simulink model "Solar_pressure_on_10_faces"  (R2023b)
settings: Solver=VariableStepAuto  StartTime=0.0  StopTime=10.0  RelTol=1e-3
undefined symbols (not defined in the file or in its folder): A_1, A_10, A_2, A_3, A_4, A_5, A_6, A_7, A_8, A_9, N_1, N_10, N_2, N_3, N_4, N_5, N_6, N_7, N_8, N_9, r_1, r_10, r_2, r_3, r_4, r_5, r_6, r_7, r_8, r_9, rho_d1, rho_d10, rho_d2, rho_d3, rho_d4, rho_d5, rho_d6, rho_d7, rho_d8, rho_d9, rho_s1, rho_s10, rho_s2, rho_s3, rho_s4, rho_s5, rho_s6, rho_s7, rho_s8, rho_s9
libraries: matrix_library x10
settings Model: Creator=rkomiii_masca  LastModifiedBy=rkomiii_masca

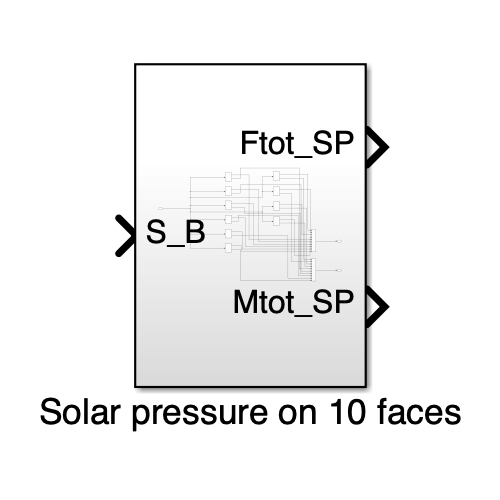
[thumbnail: Simulink's stored preview of the top-level diagram]
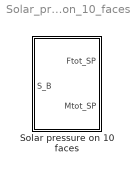
== system Solar_pressure_on_10_faces ==
  Solar pressure on 10 faces : Subsystem

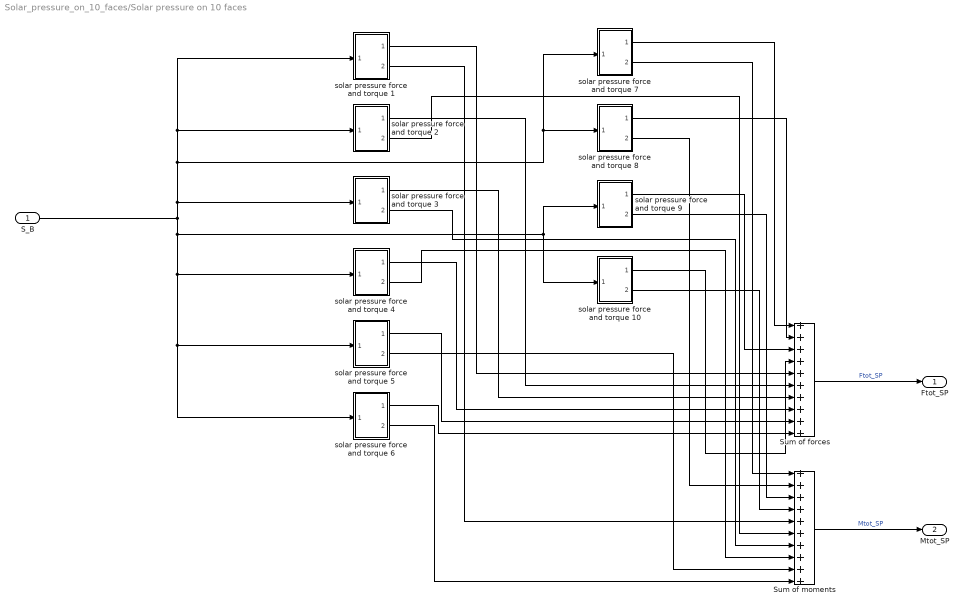
== system Solar_pressure_on_10_faces/Solar pressure on 10 faces ==
  S_B : Inport
  Sum of forces : Sum  Inputs=++++++++++
  Sum of moments : Sum  Inputs=++++++++++
  solar pressure force and torque 1 : Subsystem
  solar pressure force and torque 10 : Subsystem
  solar pressure force and torque 2 : Subsystem
  solar pressure force and torque 3 : Subsystem
  solar pressure force and torque 4 : Subsystem
  solar pressure force and torque 5 : Subsystem
  solar pressure force and torque 6 : Subsystem
  solar pressure force and torque 7 : Subsystem
  solar pressure force and torque 8 : Subsystem
  solar pressure force and torque 9 : Subsystem
  Ftot_SP : Outport
  Mtot_SP : Outport  Port=2
  wires:
  solar pressure force and torque 1/1(F_1) -> Sum of forces/5
  solar pressure force and torque 2/1(F_2) -> Sum of forces/6
  solar pressure force and torque 3/1(F_3) -> Sum of forces/7
  solar pressure force and torque 4/1(F_4) -> Sum of forces/8
  solar pressure force and torque 5/1(F_5) -> Sum of forces/9
  solar pressure force and torque 6/1(F_6) -> Sum of forces/10
  solar pressure force and torque 7/1(F_7) -> Sum of forces/1
  solar pressure force and torque 8/1(F_8) -> Sum of forces/2
  solar pressure force and torque 9/1(F_9) -> Sum of forces/3
  solar pressure force and torque 10/1(F_10) -> Sum of forces/4
  solar pressure force and torque 1/2(M_1) -> Sum of moments/5
  solar pressure force and torque 2/2(M_2) -> Sum of moments/6
  solar pressure force and torque 3/2(M_3) -> Sum of moments/7
  solar pressure force and torque 4/2(M_4) -> Sum of moments/8
  solar pressure force and torque 5/2(M_5) -> Sum of moments/9
  solar pressure force and torque 6/2(M_6) -> Sum of moments/10
  solar pressure force and torque 7/2(M_7) -> Sum of moments/1
  solar pressure force and torque 8/2(M_8) -> Sum of moments/2
  solar pressure force and torque 9/2(M_9) -> Sum of moments/3
  solar pressure force and torque 10/2(M_10) -> Sum of moments/4
  Sum of forces/1 -> Ftot_SP/1  "Ftot_SP"
  Sum of moments/1 -> Mtot_SP/1  "Mtot_SP"
  S_B/1 -> solar pressure force and torque 10/1(s_B), solar pressure force and torque 9/1(s_B), solar pressure force and torque 6/1(s_B), solar pressure force and torque 5/1(s_B), solar pressure force and torque 4/1(s_B), solar pressure force and torque 7/1(s_B), solar pressure force and torque 8/1(s_B), solar pressure force and torque 1/1(s_B), solar pressure force and torque 2/1(s_B), solar pressure force and torque 3/1(s_B)

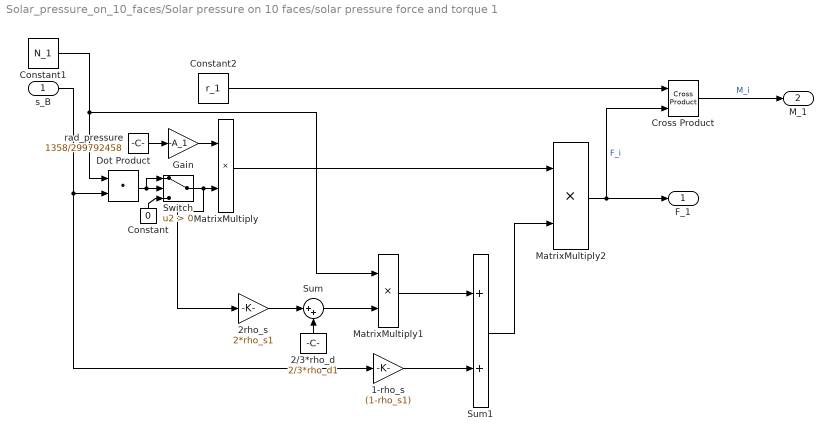
== system Solar_pressure_on_10_faces/Solar pressure on 10 faces/solar pressure force and torque 1 ==
  s_B : Inport
  1-rho_s : Gain  Gain=(1-rho_s1)
  2/3*rho_d : Constant  Value=2/3*rho_d1
  2rho_s : Gain  Gain=2*rho_s1
  Constant : Constant  Value=0
  Constant1 : Constant  Value=N_1
  Constant2 : Constant  Value=r_1
  Cross Product : matrix_library/Cross Product
  Dot Product : DotProduct  OutDataTypeStr=Inherit: Inherit via internal rule
  Gain : Gain  Gain=-A_1
  MatrixMultiply : Product
  MatrixMultiply1 : Product
  MatrixMultiply2 : Product
  Sum : Sum  Inputs=|++
  Sum1 : Sum
  Switch : Switch  Criteria=u2 > Threshold  SaturateOnIntegerOverflow=off  InputSameDT=off
  rad_pressure : Constant  Value=1358/299792458
  F_1 : Outport
  M_1 : Outport  Port=2
  wires:
  MatrixMultiply2/1 -> Cross Product/2, F_1/1  "F_i"
  MatrixMultiply/1 -> MatrixMultiply2/1
  Sum1/1 -> MatrixMultiply2/2
  s_B/1 -> 1-rho_s/1, Dot Product/2
  2rho_s/1 -> Sum/1
  1-rho_s/1 -> Sum1/2
  rad_pressure/1 -> Gain/1
  2/3*rho_d/1 -> Sum/2
  MatrixMultiply1/1 -> Sum1/1
  Constant1/1 -> MatrixMultiply1/1, Dot Product/1
  Sum/1 -> MatrixMultiply1/2
  Gain/1 -> MatrixMultiply/1
  Constant2/1 -> Cross Product/1
  Cross Product/1 -> M_1/1  "M_i"
  Dot Product/1 -> Switch/1, Switch/2
  Constant/1 -> Switch/3
  Switch/1 -> 2rho_s/1, MatrixMultiply/2

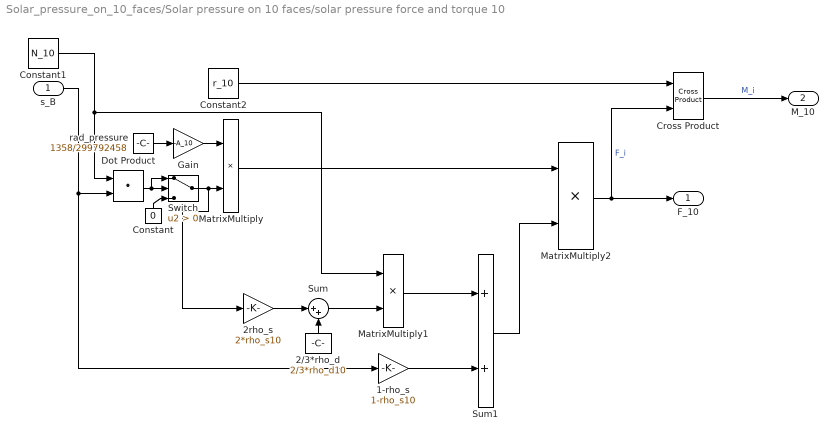
== system Solar_pressure_on_10_faces/Solar pressure on 10 faces/solar pressure force and torque 10 ==
  s_B : Inport
  1-rho_s : Gain  Gain=1-rho_s10
  2/3*rho_d : Constant  Value=2/3*rho_d10
  2rho_s : Gain  Gain=2*rho_s10
  Constant : Constant  Value=0
  Constant1 : Constant  Value=N_10
  Constant2 : Constant  Value=r_10
  Cross Product : matrix_library/Cross Product
  Dot Product : DotProduct  OutDataTypeStr=Inherit: Inherit via internal rule
  Gain : Gain  Gain=-A_10
  MatrixMultiply : Product
  MatrixMultiply1 : Product
  MatrixMultiply2 : Product
  Sum : Sum  Inputs=|++
  Sum1 : Sum
  Switch : Switch  Criteria=u2 > Threshold  SaturateOnIntegerOverflow=off  InputSameDT=off
  rad_pressure : Constant  Value=1358/299792458
  F_10 : Outport
  M_10 : Outport  Port=2
  wires:
  MatrixMultiply2/1 -> Cross Product/2, F_10/1  "F_i"
  MatrixMultiply/1 -> MatrixMultiply2/1
  Sum1/1 -> MatrixMultiply2/2
  s_B/1 -> 1-rho_s/1, Dot Product/2
  2rho_s/1 -> Sum/1
  1-rho_s/1 -> Sum1/2
  rad_pressure/1 -> Gain/1
  2/3*rho_d/1 -> Sum/2
  MatrixMultiply1/1 -> Sum1/1
  Constant1/1 -> MatrixMultiply1/1, Dot Product/1
  Sum/1 -> MatrixMultiply1/2
  Gain/1 -> MatrixMultiply/1
  Constant2/1 -> Cross Product/1
  Cross Product/1 -> M_10/1  "M_i"
  Dot Product/1 -> Switch/1, Switch/2
  Constant/1 -> Switch/3
  Switch/1 -> 2rho_s/1, MatrixMultiply/2

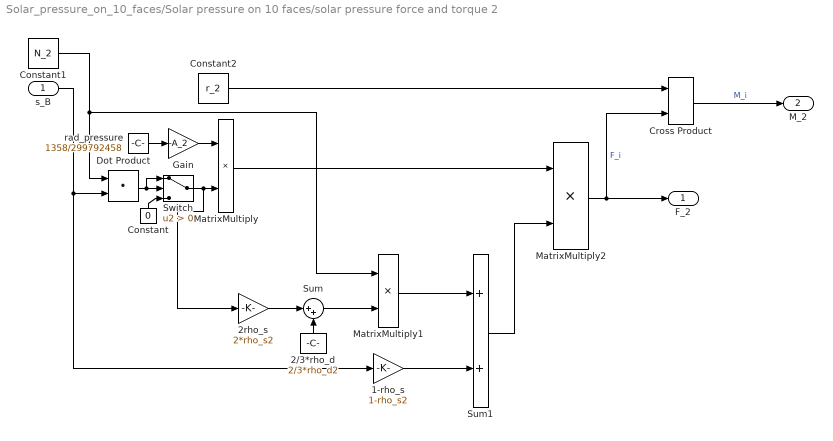
== system Solar_pressure_on_10_faces/Solar pressure on 10 faces/solar pressure force and torque 2 ==
  s_B : Inport
  1-rho_s : Gain  Gain=1-rho_s2
  2/3*rho_d : Constant  Value=2/3*rho_d2
  2rho_s : Gain  Gain=2*rho_s2
  Constant : Constant  Value=0
  Constant1 : Constant  Value=N_2
  Constant2 : Constant  Value=r_2
  Cross Product : matrix_library/Cross Product
  Dot Product : DotProduct  OutDataTypeStr=Inherit: Inherit via internal rule
  Gain : Gain  Gain=-A_2
  MatrixMultiply : Product
  MatrixMultiply1 : Product
  MatrixMultiply2 : Product
  Sum : Sum  Inputs=|++
  Sum1 : Sum
  Switch : Switch  Criteria=u2 > Threshold  SaturateOnIntegerOverflow=off  InputSameDT=off
  rad_pressure : Constant  Value=1358/299792458
  F_2 : Outport
  M_2 : Outport  Port=2
  wires:
  MatrixMultiply2/1 -> Cross Product/2, F_2/1  "F_i"
  MatrixMultiply/1 -> MatrixMultiply2/1
  Sum1/1 -> MatrixMultiply2/2
  s_B/1 -> 1-rho_s/1, Dot Product/2
  2rho_s/1 -> Sum/1
  1-rho_s/1 -> Sum1/2
  rad_pressure/1 -> Gain/1
  2/3*rho_d/1 -> Sum/2
  MatrixMultiply1/1 -> Sum1/1
  Constant1/1 -> MatrixMultiply1/1, Dot Product/1
  Sum/1 -> MatrixMultiply1/2
  Gain/1 -> MatrixMultiply/1
  Constant2/1 -> Cross Product/1
  Cross Product/1 -> M_2/1  "M_i"
  Dot Product/1 -> Switch/1, Switch/2
  Constant/1 -> Switch/3
  Switch/1 -> 2rho_s/1, MatrixMultiply/2

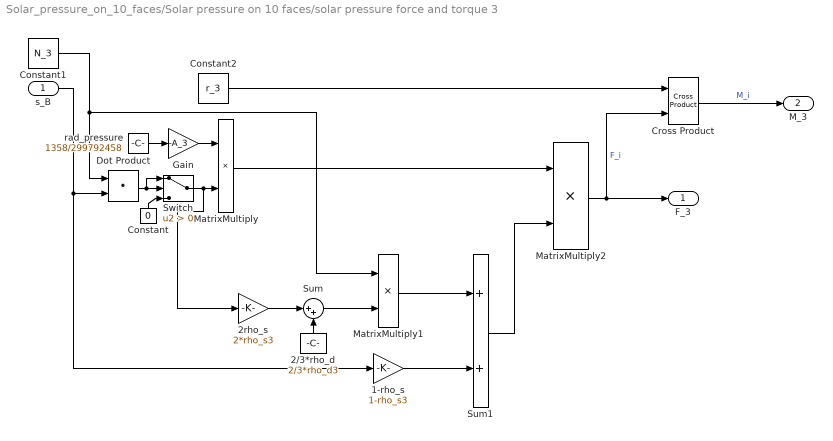
== system Solar_pressure_on_10_faces/Solar pressure on 10 faces/solar pressure force and torque 3 ==
  s_B : Inport
  1-rho_s : Gain  Gain=1-rho_s3
  2/3*rho_d : Constant  Value=2/3*rho_d3
  2rho_s : Gain  Gain=2*rho_s3
  Constant : Constant  Value=0
  Constant1 : Constant  Value=N_3
  Constant2 : Constant  Value=r_3
  Cross Product : matrix_library/Cross Product
  Dot Product : DotProduct  OutDataTypeStr=Inherit: Inherit via internal rule
  Gain : Gain  Gain=-A_3
  MatrixMultiply : Product
  MatrixMultiply1 : Product
  MatrixMultiply2 : Product
  Sum : Sum  Inputs=|++
  Sum1 : Sum
  Switch : Switch  Criteria=u2 > Threshold  SaturateOnIntegerOverflow=off  InputSameDT=off
  rad_pressure : Constant  Value=1358/299792458
  F_3 : Outport
  M_3 : Outport  Port=2
  wires:
  MatrixMultiply2/1 -> Cross Product/2, F_3/1  "F_i"
  MatrixMultiply/1 -> MatrixMultiply2/1
  Sum1/1 -> MatrixMultiply2/2
  s_B/1 -> 1-rho_s/1, Dot Product/2
  2rho_s/1 -> Sum/1
  1-rho_s/1 -> Sum1/2
  rad_pressure/1 -> Gain/1
  2/3*rho_d/1 -> Sum/2
  MatrixMultiply1/1 -> Sum1/1
  Constant1/1 -> MatrixMultiply1/1, Dot Product/1
  Sum/1 -> MatrixMultiply1/2
  Gain/1 -> MatrixMultiply/1
  Constant2/1 -> Cross Product/1
  Cross Product/1 -> M_3/1  "M_i"
  Dot Product/1 -> Switch/1, Switch/2
  Constant/1 -> Switch/3
  Switch/1 -> 2rho_s/1, MatrixMultiply/2

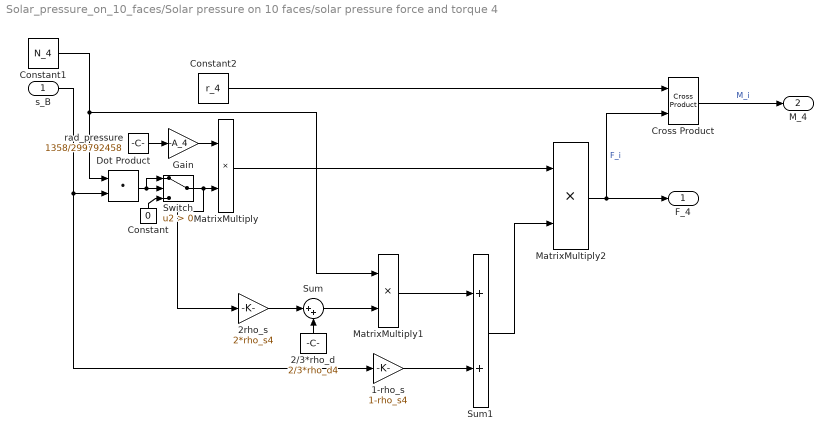
== system Solar_pressure_on_10_faces/Solar pressure on 10 faces/solar pressure force and torque 4 ==
  s_B : Inport
  1-rho_s : Gain  Gain=1-rho_s4
  2/3*rho_d : Constant  Value=2/3*rho_d4
  2rho_s : Gain  Gain=2*rho_s4
  Constant : Constant  Value=0
  Constant1 : Constant  Value=N_4
  Constant2 : Constant  Value=r_4
  Cross Product : matrix_library/Cross Product
  Dot Product : DotProduct  OutDataTypeStr=Inherit: Inherit via internal rule
  Gain : Gain  Gain=-A_4
  MatrixMultiply : Product
  MatrixMultiply1 : Product
  MatrixMultiply2 : Product
  Sum : Sum  Inputs=|++
  Sum1 : Sum
  Switch : Switch  Criteria=u2 > Threshold  SaturateOnIntegerOverflow=off  InputSameDT=off
  rad_pressure : Constant  Value=1358/299792458
  F_4 : Outport
  M_4 : Outport  Port=2
  wires:
  MatrixMultiply2/1 -> Cross Product/2, F_4/1  "F_i"
  MatrixMultiply/1 -> MatrixMultiply2/1
  Sum1/1 -> MatrixMultiply2/2
  s_B/1 -> 1-rho_s/1, Dot Product/2
  2rho_s/1 -> Sum/1
  1-rho_s/1 -> Sum1/2
  rad_pressure/1 -> Gain/1
  2/3*rho_d/1 -> Sum/2
  MatrixMultiply1/1 -> Sum1/1
  Constant1/1 -> MatrixMultiply1/1, Dot Product/1
  Sum/1 -> MatrixMultiply1/2
  Gain/1 -> MatrixMultiply/1
  Constant2/1 -> Cross Product/1
  Cross Product/1 -> M_4/1  "M_i"
  Dot Product/1 -> Switch/1, Switch/2
  Constant/1 -> Switch/3
  Switch/1 -> 2rho_s/1, MatrixMultiply/2

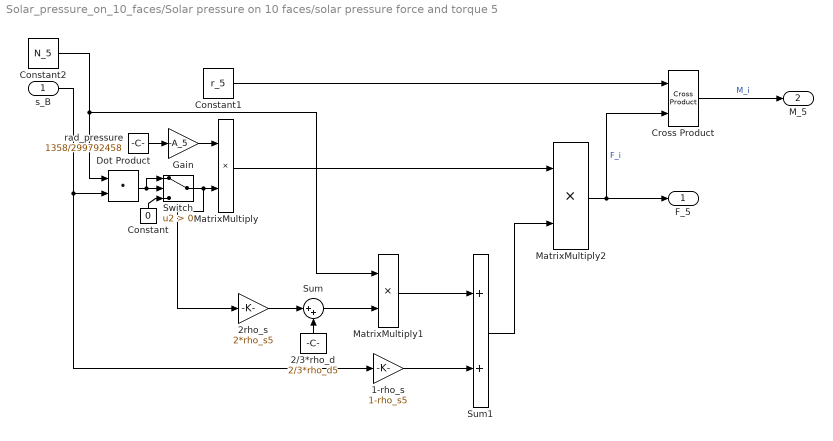
== system Solar_pressure_on_10_faces/Solar pressure on 10 faces/solar pressure force and torque 5 ==
  s_B : Inport
  1-rho_s : Gain  Gain=1-rho_s5
  2/3*rho_d : Constant  Value=2/3*rho_d5
  2rho_s : Gain  Gain=2*rho_s5
  Constant : Constant  Value=0
  Constant1 : Constant  Value=r_5
  Constant2 : Constant  Value=N_5
  Cross Product : matrix_library/Cross Product
  Dot Product : DotProduct  OutDataTypeStr=Inherit: Inherit via internal rule
  Gain : Gain  Gain=-A_5
  MatrixMultiply : Product
  MatrixMultiply1 : Product
  MatrixMultiply2 : Product
  Sum : Sum  Inputs=|++
  Sum1 : Sum
  Switch : Switch  Criteria=u2 > Threshold  SaturateOnIntegerOverflow=off  InputSameDT=off
  rad_pressure : Constant  Value=1358/299792458
  F_5 : Outport
  M_5 : Outport  Port=2
  wires:
  MatrixMultiply2/1 -> Cross Product/2, F_5/1  "F_i"
  MatrixMultiply/1 -> MatrixMultiply2/1
  Sum1/1 -> MatrixMultiply2/2
  s_B/1 -> 1-rho_s/1, Dot Product/2
  2rho_s/1 -> Sum/1
  1-rho_s/1 -> Sum1/2
  rad_pressure/1 -> Gain/1
  2/3*rho_d/1 -> Sum/2
  MatrixMultiply1/1 -> Sum1/1
  Constant2/1 -> MatrixMultiply1/1, Dot Product/1
  Sum/1 -> MatrixMultiply1/2
  Gain/1 -> MatrixMultiply/1
  Constant1/1 -> Cross Product/1
  Cross Product/1 -> M_5/1  "M_i"
  Dot Product/1 -> Switch/1, Switch/2
  Constant/1 -> Switch/3
  Switch/1 -> 2rho_s/1, MatrixMultiply/2

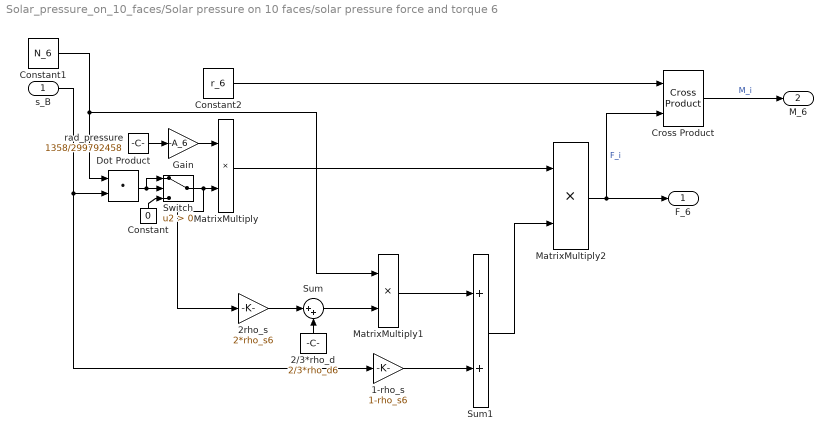
== system Solar_pressure_on_10_faces/Solar pressure on 10 faces/solar pressure force and torque 6 ==
  s_B : Inport
  1-rho_s : Gain  Gain=1-rho_s6
  2/3*rho_d : Constant  Value=2/3*rho_d6
  2rho_s : Gain  Gain=2*rho_s6
  Constant : Constant  Value=0
  Constant1 : Constant  Value=N_6
  Constant2 : Constant  Value=r_6
  Cross Product : matrix_library/Cross Product
  Dot Product : DotProduct  OutDataTypeStr=Inherit: Inherit via internal rule
  Gain : Gain  Gain=-A_6
  MatrixMultiply : Product
  MatrixMultiply1 : Product
  MatrixMultiply2 : Product
  Sum : Sum  Inputs=|++
  Sum1 : Sum
  Switch : Switch  Criteria=u2 > Threshold  SaturateOnIntegerOverflow=off  InputSameDT=off
  rad_pressure : Constant  Value=1358/299792458
  F_6 : Outport
  M_6 : Outport  Port=2
  wires:
  MatrixMultiply2/1 -> Cross Product/2, F_6/1  "F_i"
  MatrixMultiply/1 -> MatrixMultiply2/1
  Sum1/1 -> MatrixMultiply2/2
  s_B/1 -> 1-rho_s/1, Dot Product/2
  2rho_s/1 -> Sum/1
  1-rho_s/1 -> Sum1/2
  rad_pressure/1 -> Gain/1
  2/3*rho_d/1 -> Sum/2
  MatrixMultiply1/1 -> Sum1/1
  Constant1/1 -> MatrixMultiply1/1, Dot Product/1
  Sum/1 -> MatrixMultiply1/2
  Gain/1 -> MatrixMultiply/1
  Constant2/1 -> Cross Product/1
  Cross Product/1 -> M_6/1  "M_i"
  Dot Product/1 -> Switch/1, Switch/2
  Constant/1 -> Switch/3
  Switch/1 -> 2rho_s/1, MatrixMultiply/2

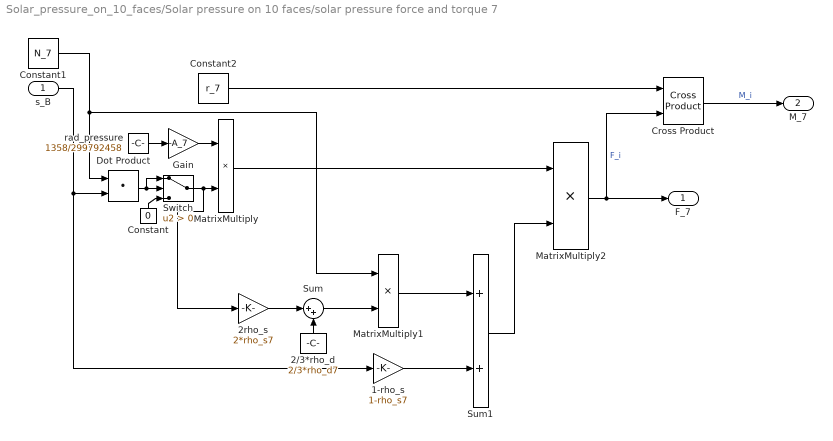
== system Solar_pressure_on_10_faces/Solar pressure on 10 faces/solar pressure force and torque 7 ==
  s_B : Inport
  1-rho_s : Gain  Gain=1-rho_s7
  2/3*rho_d : Constant  Value=2/3*rho_d7
  2rho_s : Gain  Gain=2*rho_s7
  Constant : Constant  Value=0
  Constant1 : Constant  Value=N_7
  Constant2 : Constant  Value=r_7
  Cross Product : matrix_library/Cross Product
  Dot Product : DotProduct  OutDataTypeStr=Inherit: Inherit via internal rule
  Gain : Gain  Gain=-A_7
  MatrixMultiply : Product
  MatrixMultiply1 : Product
  MatrixMultiply2 : Product
  Sum : Sum  Inputs=|++
  Sum1 : Sum
  Switch : Switch  Criteria=u2 > Threshold  SaturateOnIntegerOverflow=off  InputSameDT=off
  rad_pressure : Constant  Value=1358/299792458
  F_7 : Outport
  M_7 : Outport  Port=2
  wires:
  MatrixMultiply2/1 -> Cross Product/2, F_7/1  "F_i"
  MatrixMultiply/1 -> MatrixMultiply2/1
  Sum1/1 -> MatrixMultiply2/2
  s_B/1 -> 1-rho_s/1, Dot Product/2
  2rho_s/1 -> Sum/1
  1-rho_s/1 -> Sum1/2
  rad_pressure/1 -> Gain/1
  2/3*rho_d/1 -> Sum/2
  MatrixMultiply1/1 -> Sum1/1
  Constant1/1 -> MatrixMultiply1/1, Dot Product/1
  Sum/1 -> MatrixMultiply1/2
  Gain/1 -> MatrixMultiply/1
  Constant2/1 -> Cross Product/1
  Cross Product/1 -> M_7/1  "M_i"
  Dot Product/1 -> Switch/1, Switch/2
  Constant/1 -> Switch/3
  Switch/1 -> 2rho_s/1, MatrixMultiply/2

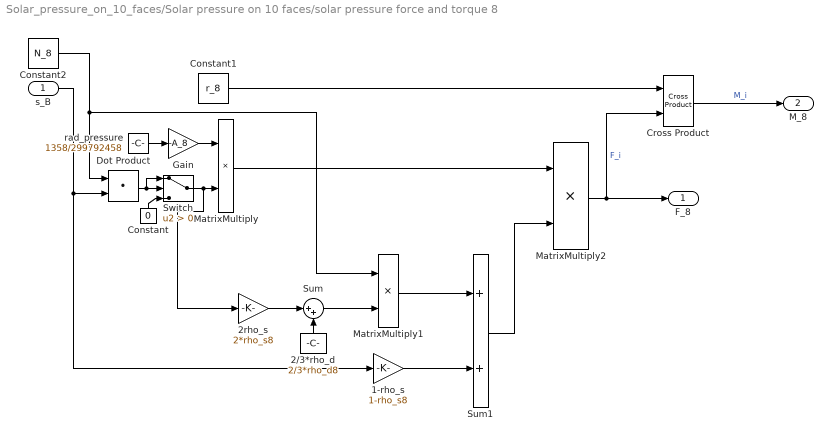
== system Solar_pressure_on_10_faces/Solar pressure on 10 faces/solar pressure force and torque 8 ==
  s_B : Inport
  1-rho_s : Gain  Gain=1-rho_s8
  2/3*rho_d : Constant  Value=2/3*rho_d8
  2rho_s : Gain  Gain=2*rho_s8
  Constant : Constant  Value=0
  Constant1 : Constant  Value=r_8
  Constant2 : Constant  Value=N_8
  Cross Product : matrix_library/Cross Product
  Dot Product : DotProduct  OutDataTypeStr=Inherit: Inherit via internal rule
  Gain : Gain  Gain=-A_8
  MatrixMultiply : Product
  MatrixMultiply1 : Product
  MatrixMultiply2 : Product
  Sum : Sum  Inputs=|++
  Sum1 : Sum
  Switch : Switch  Criteria=u2 > Threshold  SaturateOnIntegerOverflow=off  InputSameDT=off
  rad_pressure : Constant  Value=1358/299792458
  F_8 : Outport
  M_8 : Outport  Port=2
  wires:
  MatrixMultiply2/1 -> Cross Product/2, F_8/1  "F_i"
  MatrixMultiply/1 -> MatrixMultiply2/1
  Sum1/1 -> MatrixMultiply2/2
  s_B/1 -> 1-rho_s/1, Dot Product/2
  2rho_s/1 -> Sum/1
  1-rho_s/1 -> Sum1/2
  rad_pressure/1 -> Gain/1
  2/3*rho_d/1 -> Sum/2
  MatrixMultiply1/1 -> Sum1/1
  Constant2/1 -> MatrixMultiply1/1, Dot Product/1
  Sum/1 -> MatrixMultiply1/2
  Gain/1 -> MatrixMultiply/1
  Constant1/1 -> Cross Product/1
  Cross Product/1 -> M_8/1  "M_i"
  Dot Product/1 -> Switch/1, Switch/2
  Constant/1 -> Switch/3
  Switch/1 -> 2rho_s/1, MatrixMultiply/2

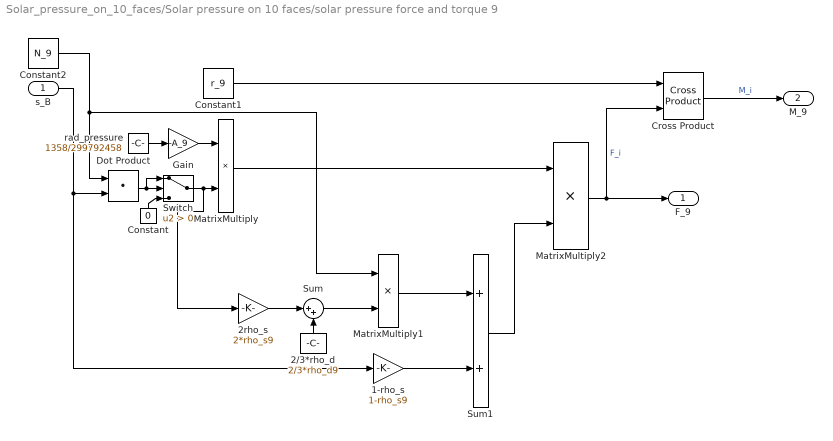
== system Solar_pressure_on_10_faces/Solar pressure on 10 faces/solar pressure force and torque 9 ==
  s_B : Inport
  1-rho_s : Gain  Gain=1-rho_s9
  2/3*rho_d : Constant  Value=2/3*rho_d9
  2rho_s : Gain  Gain=2*rho_s9
  Constant : Constant  Value=0
  Constant1 : Constant  Value=r_9
  Constant2 : Constant  Value=N_9
  Cross Product : matrix_library/Cross Product
  Dot Product : DotProduct  OutDataTypeStr=Inherit: Inherit via internal rule
  Gain : Gain  Gain=-A_9
  MatrixMultiply : Product
  MatrixMultiply1 : Product
  MatrixMultiply2 : Product
  Sum : Sum  Inputs=|++
  Sum1 : Sum
  Switch : Switch  Criteria=u2 > Threshold  SaturateOnIntegerOverflow=off  InputSameDT=off
  rad_pressure : Constant  Value=1358/299792458
  F_9 : Outport
  M_9 : Outport  Port=2
  wires:
  MatrixMultiply2/1 -> Cross Product/2, F_9/1  "F_i"
  MatrixMultiply/1 -> MatrixMultiply2/1
  Sum1/1 -> MatrixMultiply2/2
  s_B/1 -> 1-rho_s/1, Dot Product/2
  2rho_s/1 -> Sum/1
  1-rho_s/1 -> Sum1/2
  rad_pressure/1 -> Gain/1
  2/3*rho_d/1 -> Sum/2
  MatrixMultiply1/1 -> Sum1/1
  Constant2/1 -> MatrixMultiply1/1, Dot Product/1
  Sum/1 -> MatrixMultiply1/2
  Gain/1 -> MatrixMultiply/1
  Constant1/1 -> Cross Product/1
  Cross Product/1 -> M_9/1  "M_i"
  Dot Product/1 -> Switch/1, Switch/2
  Constant/1 -> Switch/3
  Switch/1 -> 2rho_s/1, MatrixMultiply/2
